simulink model "Drone_Simulation"  (R2020a)
settings: Solver=ode1  StartTime=0.0  StopTime=15  FixedStep=1e-3
undefined symbols (not defined in the file): AeEMSC, alpha1TDDBSC, B, bBNG, bEMSC, bEVCAP, BNG_Motor1, BNG_Motor2, BNG_Motor3, BNG_Motor4, BNG_Motor5, BNG_Motor6, bp, bq, br, bTDDBSC, bWDG, C_A, C_mot, C_th_esc, CAPEV_Motor1, CAPEV_Motor2, CAPEV_Motor3, CAPEV_Motor4, CAPEV_Motor5, CAPEV_Motor6, cdx, cdy, cdz, EaEMSC, EaEVCAP, EalphaTDDBSC, EaTDDBSC, EaWDG, FuselageContactForces, g, JrefEMSC, k_b, Kp, Kp2, Kq, Kq2, Kr, Kr2, kv, Kx, Ky, Kz, Kz2, LeftAftArm, LeftAftSkid, LeftArm, LeftFrontArm, LeftFrontSkid, LeftSideContactForces, LnomEMSC, LnomEVCAP, LnomTDDBSC, LnomWDG, Lower ... (+65)
libraries: sm_lib x90, nesl_utility x76, fl_lib x59, ee_lib x18, batteryecm_lib x2, dspinverses x1, dspmtrx3 x1
(part 5 of 5)

== system Drone_Simulation/PLANT MODEL/ELECTRIC SYSTEM/Motor 2/RPM to Resistive Torque and Thrust ==
  Angular Speed : Inport
  Gain : Gain  Gain=-1
  Math Function : Math  Operator=square  SaturateOnIntegerOverflow=on
  Math Function1 : Math  Operator=square  SaturateOnIntegerOverflow=on
  Math Function2 : Math  Operator=square  SaturateOnIntegerOverflow=on
  Square Root : Sqrt  SaturateOnIntegerOverflow=on
  Sum : Sum  Inputs=+++
  Thrust & Torque Based on Propeller Rotational and Translational Velocity : MATLAB Function  TreatAsAtomicUnit=on
  Thrust : Outport
  Resistive Torque : Outport  Port=2
  wires:
  Gain/1 -> Resistive Torque/1
  Thrust & Torque Based on Propeller Rotational and Translational Velocity/2(Torque) -> Gain/1
  Angular Speed/1 -> Thrust & Torque Based on Propeller Rotational and Translational Velocity/2(RPM)  "Speed"
  Thrust & Torque Based on Propeller Rotational and Translational Velocity/1(Thrust) -> Thrust/1
  [DX] -> Math Function/1
  Math Function/1 -> Sum/1
  Math Function2/1 -> Sum/3
  Sum/1 -> Square Root/1
  Math Function1/1 -> Sum/2
  [DZ] -> Math Function2/1
  [DY] -> Math Function1/1
  Square Root/1 -> Thrust & Torque Based on Propeller Rotational and Translational Velocity/1(Velocity)

== system Drone_Simulation/PLANT MODEL/ELECTRIC SYSTEM/Motor 3/RPM to Resistive Torque and Thrust ==
  Angular Speed : Inport
  Gain : Gain  Gain=-1
  Math Function : Math  Operator=square  SaturateOnIntegerOverflow=on
  Math Function1 : Math  Operator=square  SaturateOnIntegerOverflow=on
  Math Function2 : Math  Operator=square  SaturateOnIntegerOverflow=on
  Square Root : Sqrt  SaturateOnIntegerOverflow=on
  Sum : Sum  Inputs=+++
  Thrust & Torque Based on Propeller Rotational and Translational Velocity : MATLAB Function  TreatAsAtomicUnit=on
  Thrust : Outport
  Resistive Torque : Outport  Port=2
  wires:
  Gain/1 -> Resistive Torque/1
  Thrust & Torque Based on Propeller Rotational and Translational Velocity/2(Torque) -> Gain/1
  Angular Speed/1 -> Thrust & Torque Based on Propeller Rotational and Translational Velocity/2(RPM)  "Speed"
  Thrust & Torque Based on Propeller Rotational and Translational Velocity/1(Thrust) -> Thrust/1
  [DX] -> Math Function/1
  Math Function/1 -> Sum/1
  Math Function2/1 -> Sum/3
  Sum/1 -> Square Root/1
  Square Root/1 -> Thrust & Torque Based on Propeller Rotational and Translational Velocity/1(Velocity)
  Math Function1/1 -> Sum/2
  [DZ] -> Math Function2/1
  [DY] -> Math Function1/1

== system Drone_Simulation/PLANT MODEL/ELECTRIC SYSTEM/Motor 4/RPM to Resistive Torque and Thrust ==
  Angular Speed : Inport
  Gain : Gain  Gain=-1
  Math Function : Math  Operator=square  SaturateOnIntegerOverflow=on
  Math Function1 : Math  Operator=square  SaturateOnIntegerOverflow=on
  Math Function2 : Math  Operator=square  SaturateOnIntegerOverflow=on
  Square Root : Sqrt  SaturateOnIntegerOverflow=on
  Sum : Sum  Inputs=+++
  Thrust & Torque Based on Propeller Rotational and Translational Velocity : MATLAB Function  TreatAsAtomicUnit=on
  Thrust : Outport
  Resistive Torque : Outport  Port=2
  wires:
  Gain/1 -> Resistive Torque/1
  Thrust & Torque Based on Propeller Rotational and Translational Velocity/2(Torque) -> Gain/1
  Angular Speed/1 -> Thrust & Torque Based on Propeller Rotational and Translational Velocity/2(RPM)  "Speed"
  Thrust & Torque Based on Propeller Rotational and Translational Velocity/1(Thrust) -> Thrust/1
  [DX] -> Math Function/1
  Math Function/1 -> Sum/1
  Math Function2/1 -> Sum/3
  Sum/1 -> Square Root/1
  Square Root/1 -> Thrust & Torque Based on Propeller Rotational and Translational Velocity/1(Velocity)
  Math Function1/1 -> Sum/2
  [DZ] -> Math Function2/1
  [DY] -> Math Function1/1

== system Drone_Simulation/PLANT MODEL/ELECTRIC SYSTEM/Motor 5/RPM to Resistive Torque and Thrust ==
  Angular Speed : Inport
  Gain : Gain  Gain=-1
  Math Function : Math  Operator=square  SaturateOnIntegerOverflow=on
  Math Function1 : Math  Operator=square  SaturateOnIntegerOverflow=on
  Math Function2 : Math  Operator=square  SaturateOnIntegerOverflow=on
  Square Root : Sqrt  SaturateOnIntegerOverflow=on
  Sum : Sum  Inputs=+++
  Thrust & Torque Based on Propeller Rotational and Translational Velocity : MATLAB Function  TreatAsAtomicUnit=on
  Thrust : Outport
  Resistive Torque : Outport  Port=2
  wires:
  Gain/1 -> Resistive Torque/1
  Thrust & Torque Based on Propeller Rotational and Translational Velocity/2(Torque) -> Gain/1
  Angular Speed/1 -> Thrust & Torque Based on Propeller Rotational and Translational Velocity/2(RPM)  "Speed"
  Thrust & Torque Based on Propeller Rotational and Translational Velocity/1(Thrust) -> Thrust/1
  [DX] -> Math Function/1
  Math Function/1 -> Sum/1
  Math Function2/1 -> Sum/3
  Sum/1 -> Square Root/1
  Square Root/1 -> Thrust & Torque Based on Propeller Rotational and Translational Velocity/1(Velocity)
  Math Function1/1 -> Sum/2
  [DZ] -> Math Function2/1
  [DY] -> Math Function1/1

== system Drone_Simulation/PLANT MODEL/ELECTRIC SYSTEM/Motor 6/RPM to Resistive Torque and Thrust ==
  Angular Speed : Inport
  Gain : Gain  Gain=-1
  Math Function : Math  Operator=square  SaturateOnIntegerOverflow=on
  Math Function1 : Math  Operator=square  SaturateOnIntegerOverflow=on
  Math Function2 : Math  Operator=square  SaturateOnIntegerOverflow=on
  Square Root : Sqrt  SaturateOnIntegerOverflow=on
  Sum : Sum  Inputs=+++
  Thrust & Torque Based on Propeller Rotational and Translational Velocity : MATLAB Function  TreatAsAtomicUnit=on
  Thrust : Outport
  Resistive Torque : Outport  Port=2
  wires:
  Gain/1 -> Resistive Torque/1
  Thrust & Torque Based on Propeller Rotational and Translational Velocity/2(Torque) -> Gain/1
  Angular Speed/1 -> Thrust & Torque Based on Propeller Rotational and Translational Velocity/2(RPM)  "Speed"
  Thrust & Torque Based on Propeller Rotational and Translational Velocity/1(Thrust) -> Thrust/1
  [DX] -> Math Function/1
  Math Function/1 -> Sum/1
  Math Function2/1 -> Sum/3
  Sum/1 -> Square Root/1
  Square Root/1 -> Thrust & Torque Based on Propeller Rotational and Translational Velocity/1(Velocity)
  Math Function1/1 -> Sum/2
  [DZ] -> Math Function2/1
  [DY] -> Math Function1/1

== system Drone_Simulation/PLANT MODEL/SENSORS/Quaternion to Rotation Angles, XYZ order/If Action Subsystem ==
  Action Port : ActionPort  ActionPortLabel=if(u1 > 1)
  Constant : Constant  SampleTime=-1
  OutputPos1 : Outport  InitialOutput=0  VectorParamsAs1DForOutWhenUnconnected=off
  wires:
  Constant/1 -> OutputPos1/1

== system Drone_Simulation/PLANT MODEL/SENSORS/Quaternion to Rotation Angles, XYZ order/If Action Subsystem1 ==
  Action Port : ActionPort  ActionPortLabel=elseif(u1 < -1)
  Constant : Constant  SampleTime=-1
  OutputNeg1 : Outport  InitialOutput=0  VectorParamsAs1DForOutWhenUnconnected=off
  wires:
  Constant/1 -> OutputNeg1/1

== system Drone_Simulation/PLANT MODEL/SENSORS/Quaternion to Rotation Angles, XYZ order/If Action Subsystem2 ==
  In : Inport
  Action Port : ActionPort  ActionPortLabel=else
  OutOrig : Outport  InitialOutput=0  VectorParamsAs1DForOutWhenUnconnected=off
  wires:
  In/1 -> OutOrig/1

== matlab function Drone_Simulation/PLANT MODEL/ELECTRIC SYSTEM/Motor 4/RPM to Resistive Torque and Thrust/Thrust & Torque Based on Propeller Rotational and Translational Velocity ==
  data: Thrust output; Velocity input; RPM input; Torque output
function [Thrust,Torque]= fcn(Velocity, RPM)

%Thrust

s1 = 0.007241;
s2 = -7.12e-05;
s3 = -0.00219;
s4 = -1.683e-05;
s5 = 1.619e-07;
Thrust = s1*Velocity + s2*RPM + s3*Velocity.^2 + s4*Velocity.*RPM + s5*RPM.^2;

%Torque

k1 = 0.000295;
k2 = -1.33e-07;
k3 = -7.089e-05;
k4 = 7.352e-08;
k5 = 2.21e-09;
Torque = k1*Velocity + k2*RPM + k3*Velocity.^2 + k4*Velocity.*RPM + k5*RPM.^2;

== matlab function Drone_Simulation/PLANT MODEL/ELECTRIC SYSTEM/Motor 5/RPM to Resistive Torque and Thrust/Thrust & Torque Based on Propeller Rotational and Translational Velocity ==
  data: Thrust output; Velocity input; RPM input; Torque output
function [Thrust,Torque]= fcn(Velocity, RPM)

%Thrust

s1 = 0.007241;
s2 = -7.12e-05;
s3 = -0.00219;
s4 = -1.683e-05;
s5 = 1.619e-07;
Thrust = s1*Velocity + s2*RPM + s3*Velocity.^2 + s4*Velocity.*RPM + s5*RPM.^2;

%Torque

k1 = 0.000295;
k2 = -1.33e-07;
k3 = -7.089e-05;
k4 = 7.352e-08;
k5 = 2.21e-09;
Torque = k1*Velocity + k2*RPM + k3*Velocity.^2 + k4*Velocity.*RPM + k5*RPM.^2;

== matlab function Drone_Simulation/PLANT MODEL/ELECTRIC SYSTEM/Motor 2/RPM to Resistive Torque and Thrust/Thrust & Torque Based on Propeller Rotational and Translational Velocity ==
  data: Thrust output; Velocity input; RPM input; Torque output
function [Thrust,Torque]= fcn(Velocity, RPM)

%Thrust

s1 = 0.007241;
s2 = -7.12e-05;
s3 = -0.00219;
s4 = -1.683e-05;
s5 = 1.619e-07;
Thrust = s1*Velocity + s2*RPM + s3*Velocity.^2 + s4*Velocity.*RPM + s5*RPM.^2;

%Torque

k1 = 0.000295;
k2 = -1.33e-07;
k3 = -7.089e-05;
k4 = 7.352e-08;
k5 = 2.21e-09;
Torque = k1*Velocity + k2*RPM + k3*Velocity.^2 + k4*Velocity.*RPM + k5*RPM.^2;

== matlab function Drone_Simulation/PLANT MODEL/ELECTRIC SYSTEM/Motor 6/RPM to Resistive Torque and Thrust/Thrust & Torque Based on Propeller Rotational and Translational Velocity ==
  data: Thrust output; Velocity input; RPM input; Torque output
function [Thrust,Torque]= fcn(Velocity, RPM)

%Thrust

s1 = 0.007241;
s2 = -7.12e-05;
s3 = -0.00219;
s4 = -1.683e-05;
s5 = 1.619e-07;
Thrust = s1*Velocity + s2*RPM + s3*Velocity.^2 + s4*Velocity.*RPM + s5*RPM.^2;

%Torque

k1 = 0.000295;
k2 = -1.33e-07;
k3 = -7.089e-05;
k4 = 7.352e-08;
k5 = 2.21e-09;
Torque = k1*Velocity + k2*RPM + k3*Velocity.^2 + k4*Velocity.*RPM + k5*RPM.^2;

== matlab function Drone_Simulation/PLANT MODEL/ELECTRIC SYSTEM/Motor 3/RPM to Resistive Torque and Thrust/Thrust & Torque Based on Propeller Rotational and Translational Velocity ==
  data: Thrust output; Velocity input; RPM input; Torque output
function [Thrust,Torque]= fcn(Velocity, RPM)

%Thrust

s1 = 0.007241;
s2 = -7.12e-05;
s3 = -0.00219;
s4 = -1.683e-05;
s5 = 1.619e-07;
Thrust = s1*Velocity + s2*RPM + s3*Velocity.^2 + s4*Velocity.*RPM + s5*RPM.^2;

%Torque

k1 = 0.000295;
k2 = -1.33e-07;
k3 = -7.089e-05;
k4 = 7.352e-08;
k5 = 2.21e-09;
Torque = k1*Velocity + k2*RPM + k3*Velocity.^2 + k4*Velocity.*RPM + k5*RPM.^2;

== matlab function Drone_Simulation/Trajectory/Trajectory Control ==
  settings: updateMethod=DISCRETE
  data: xPosition output; missionPlanX input; missionPlanY input; missionPlanZ input; missionPlanYaw input; timeConstant input; yPosition output; zPosition output; simulationTime input; yaw output
function [xPosition, yPosition, zPosition, yaw] = fcn(missionPlanX, missionPlanY, missionPlanZ, missionPlanYaw, timeConstant, simulationTime)
    persistent prevX prevY prevZ prevYaw index startTime
    if isempty(prevX)
        % Initialize the previous position, yaw, index, and timer variables
        prevX = missionPlanX(1);
        prevY = missionPlanY(1);
        prevZ = missionPlanZ(1);
        prevYaw = missionPlanYaw(1);
        index = 1;
        startTime = simulationTime;  % Record the start time
    end
    
    % Get the number of points in the mission plan
    numPoints = numel(missionPlanX);
    
    % Wrap the index within the valid range of the mission plan matrices
    if index > numPoints
        % Output the last position and yaw as signals
        xPosition = prevX;
        yPosition = prevY;
        zPosition = prevZ;
        yaw = prevYaw;
        return; % Exit the function
    end
    
    % Get the current position and yaw from the mission plan matrices
    currX = missionPlanX(index);
    currY = missionPlanY(index);
    currZ = missionPlanZ(index);
    currYaw = missionPlanYaw(index);
    
    % Calculate the Euclidean distance
    distance = sqrt((currX - prevX)^2 + (currY - prevY)^2 + (currZ - prevZ)^2+(currYaw - prevYaw)^2);
    
    % Calculate the delay time
    delay = distance * timeConstant;
    
    % Check if the elapsed time is less than the scaled delay
    elapsedTime = simulationTime - startTime;
    
    if elapsedTime < delay
        % Output the previous position and yaw as long as the delay is not reached
        xPosition = prevX;
        yPosition = prevY;
        zPosition = prevZ;
        yaw = prevYaw;
    else
        % Update the previous position and yaw
        prevX = currX;
        prevY = currY;
        prevZ = currZ;
        prevYaw = currYaw;
        
        % Update the index for the next point
        index = index + 1;
        
        % Reset the start time for the next delay
        startTime = simulationTime;
        
        % Output the current position and yaw
        xPosition = currX;
        yPosition = currY;
        zPosition = currZ;
        yaw = currYaw;
    end
end

== matlab function Drone_Simulation/PLANT MODEL/ELECTRIC SYSTEM/Motor 1/RPM to Resistive Torque and Thrust1/Thrust & Torque Based on Propeller Rotational and Translational Velocity ==
  data: Thrust output; Velocity input; RPM input; Torque output
function [Thrust,Torque]= fcn(Velocity, RPM)

%Thrust

s1 = 0.007241;
s2 = -7.12e-05;
s3 = -0.00219;
s4 = -1.683e-05;
s5 = 1.619e-07;
Thrust = s1*Velocity + s2*RPM + s3*Velocity.^2 + s4*Velocity.*RPM + s5*RPM.^2;

%Torque

k1 = 0.000295;
k2 = -1.33e-07;
k3 = -7.089e-05;
k4 = 7.352e-08;
k5 = 2.21e-09;
Torque = k1*Velocity + k2*RPM + k3*Velocity.^2 + k4*Velocity.*RPM + k5*RPM.^2;
